simulink model "springDampMass"  (R2021a)
settings: Solver=VariableStepAuto  StartTime=0.0  StopTime=10  FixedStep=10^-2  RelTol=1e-3
model workspace (MAT data in the model file):
  K = 497.616525424
  M = 5
  d = 20.1947463768
libraries: fl_lib x12, nesl_utility x5
settings Model: EnablePacing=on  PacingRate=0.500000  Creator=ditde  LastModifiedBy=ditde

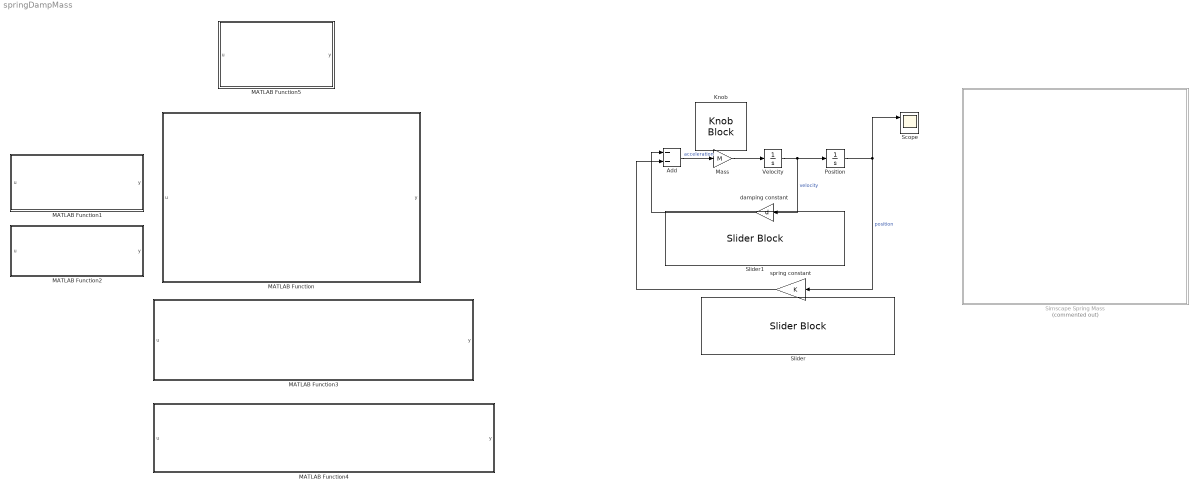
== system springDampMass ==
  Add : Sum  Inputs=--
  Knob : KnobBlock  ScaleMax=5
  MATLAB Function : MATLAB Function  TreatAsAtomicUnit=on
  MATLAB Function1 : MATLAB Function  TreatAsAtomicUnit=on
  MATLAB Function2 : MATLAB Function  TreatAsAtomicUnit=on
  MATLAB Function3 : MATLAB Function  TreatAsAtomicUnit=on
  MATLAB Function4 : MATLAB Function  TreatAsAtomicUnit=on
  MATLAB Function5 : MATLAB Function  TreatAsAtomicUnit=on
  Mass : Gain  Gain=M
  Position : Integrator  InitialCondition=1
  Scope : Scope  NumInputPorts=3
  Simscape Spring Mass : Subsystem  Commented=on
  Slider : SliderBlock  LabelPosition=Bottom  ScaleMax=1000
  Slider1 : SliderBlock  LabelPosition=Hide
  Velocity : Integrator
  damping constant : Gain  Gain=d
  spring constant : Gain  Gain=K
  wires:
  Mass/1 -> Velocity/1
  Velocity/1 -> damping constant/1, Position/1  "velocity"
  Position/1 -> Scope/1, spring constant/1  "position"
  Add/1 -> Mass/1  "acceleration"
  damping constant/1 -> Add/1
  spring constant/1 -> Add/2

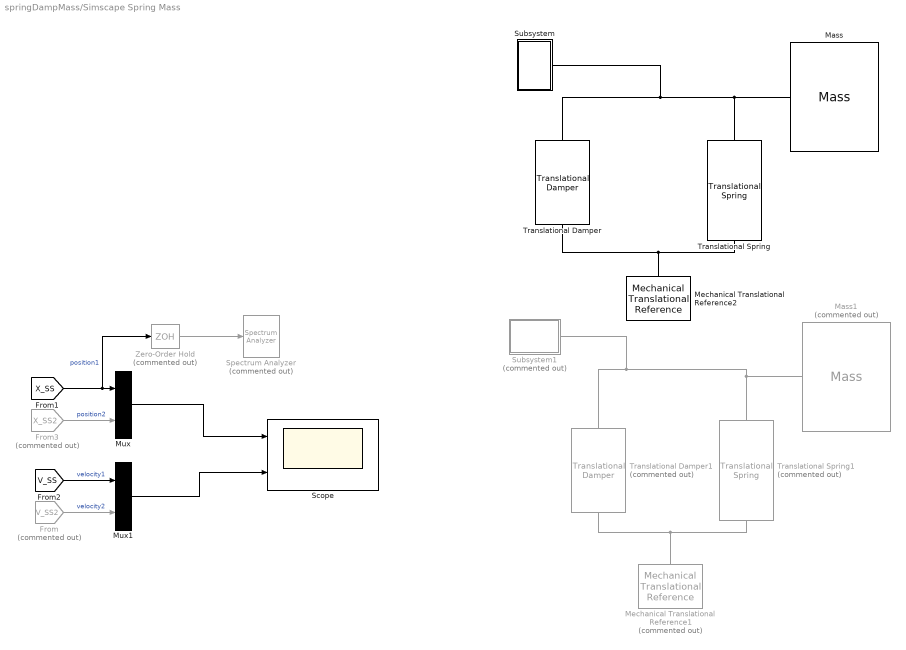
== system springDampMass/Simscape Spring Mass ==
  From : From  Commented=on  GotoTag=V_SS2  TagVisibility=global
  From3 : From  Commented=on  GotoTag=X_SS2  TagVisibility=global
  Mass : fl_lib/Mechanical/Translational Elements/Mass  mass=M kg  num_ports=foundation.enum.numPorts2.one  v_specify=off  v_priority=High  v=0 m/s  v_nominal_specify=off  v_nominal_unit=m/s  v_nominal_value=1  f_specify=off  f_priority=None  f=0 N  f_nominal_specify=off  f_nominal_unit=N  f_nominal_value=1
  Mass1 : fl_lib/Mechanical/Translational Elements/Mass  Commented=on  mass=4.1 kg  num_ports=foundation.enum.numPorts2.one  v_specify=off  v_priority=High  v=0 m/s  v_nominal_specify=off  v_nominal_unit=m/s  v_nominal_value=1  f_specify=off  f_priority=None  f=0 N  f_nominal_specify=off  f_nominal_unit=N  f_nominal_value=1
  Mechanical Translational Reference1 : fl_lib/Mechanical/Translational Elements/Mechanical Translational Reference  Commented=on
  Mechanical Translational Reference2 : fl_lib/Mechanical/Translational Elements/Mechanical Translational Reference
  Mux : Mux  Inputs=2
  Mux1 : Mux  Inputs=2
  Scope : Scope  NumInputPorts=2
  Spectrum Analyzer : SpectrumAnalyzer  Commented=on
  Subsystem : Subsystem
  Subsystem1 : Subsystem  Commented=on
      settings: PortSchema="{\"entries\":[{\"content\":{\"sides\":[{\"content\":{\"connectorIds\":[]},\"type\":\"ConnectorPlacement.EquallySpacedRectSide\",\"uuid\":\"3b3e8523-10d3-43b9-9f77-b9b637dbc56d\"},{\"content\":{\"connectorIds\":[],\"side\":\"RIGHT\"},\"type\":\"ConnectorPlacement.EquallySpacedRectSide\",\"uuid\":\"46eb001f-7b0b-4a31-ad1e-86922fc41839\"},{\"content\":{\"connectorIds\":[],\"side\":\"TOP\"},\"type\":\"ConnectorPlacement.EquallySpacedRectSide\",\"uuid\":\"e7c34988-a452-46fb-a57a-78d1edee4f1a\"},{\"content\":{\"connectorIds\":[\"RConn1\"],\"side\":\"BOTTOM\"},\"type\":\"ConnectorPlacement.EquallySpacedRectSide\",\"uuid\":\"a95b3fbc-c6ac-47a7-9bde-b25b780e38b5\"}]},\"type\":\"ConnectorPlacement.EquallySpacedConnector\",\"uuid\":\"dd414060-0bc3-4aae-86f3-2c1761549555\"}],\"packageUris\":[\"http://schema.mathworks.com/mf0/Connector/R2020b\"],\"version\":\"1.0\"}"
  Translational Damper : fl_lib/Mechanical/Translational Elements/Translational Damper  D=d N/(m/s)  v_specify=off  v_priority=None  v=0 m/s  v_nominal_specify=off  v_nominal_unit=m/s  v_nominal_value=1  f_specify=off  f_priority=None  f=1 N  f_nominal_specify=off  f_nominal_unit=N  f_nominal_value=1
  Translational Damper1 : fl_lib/Mechanical/Translational Elements/Translational Damper  Commented=on  D=0 N/(m/s)  v_specify=off  v_priority=None  v=0 m/s  v_nominal_specify=off  v_nominal_unit=m/s  v_nominal_value=1  f_specify=off  f_priority=None  f=1 N  f_nominal_specify=off  f_nominal_unit=N  f_nominal_value=1
  Translational Spring : fl_lib/Mechanical/Translational Elements/Translational Spring  spr_rate=K N/m  v_specify=off  v_priority=None  v=0 m/s  v_nominal_specify=off  v_nominal_unit=m/s  v_nominal_value=1  f_specify=off  f_priority=None  f=0 N  f_nominal_specify=off  f_nominal_unit=N  f_nominal_value=1  x_specify=on  x_priority=High  x=1 m  x_nominal_specify=off  x_nominal_unit=m  x_nominal_value=1
  Translational Spring1 : fl_lib/Mechanical/Translational Elements/Translational Spring  Commented=on  spr_rate=456 N/m  v_specify=off  v_priority=None  v=0 m/s  v_nominal_specify=off  v_nominal_unit=m/s  v_nominal_value=1  f_specify=off  f_priority=None  f=0 N  f_nominal_specify=off  f_nominal_unit=N  f_nominal_value=1  x_specify=on  x_priority=High  x=1 m  x_nominal_specify=off  x_nominal_unit=m  x_nominal_value=1
  Zero-Order Hold : ZeroOrderHold  Commented=on  SampleTime=-1
  wires:
  [X_SS] -> Zero-Order Hold/1, Mux/1  "position1"
  Zero-Order Hold/1 -> Spectrum Analyzer/1
  Mux/1 -> Scope/1
  From/1 -> Mux1/2  "velocity2"
  From3/1 -> Mux/2  "position2"
  Mux1/1 -> Scope/2
  [V_SS] -> Mux1/1  "velocity1"
  connections:
  Mass1/LConn1 -- Subsystem1/RConn1 -- Translational Damper1/LConn1 -- Translational Spring1/LConn1
  Mass/LConn1 -- Translational Damper/LConn1 -- Subsystem/LConn1 -- Translational Spring/LConn1
  Translational Damper1/RConn1 -- Translational Spring1/RConn1 -- Mechanical Translational Reference1/LConn1
  Translational Damper/RConn1 -- Mechanical Translational Reference2/LConn1 -- Translational Spring/RConn1

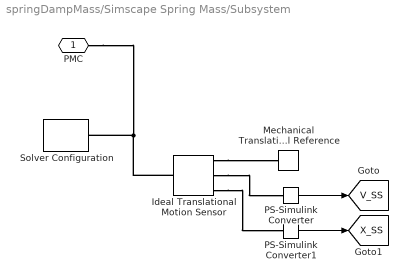
== system springDampMass/Simscape Spring Mass/Subsystem ==
  Ideal Translational Motion Sensor : fl_lib/Mechanical/Mechanical Sensors/Ideal Translational Motion Sensor  offset=1 m
  Mechanical Translational Reference : fl_lib/Mechanical/Translational Elements/Mechanical Translational Reference
  PS-Simulink Converter : nesl_utility/PS-Simulink Converter  PhysicalDomain=network_engine_domain  SubClassName=ps_output  LeftPortType=input  RightPortType=output  PseudoPeriodic=off  Frequencies=[]  Unit=inherit  AffineConversion=off
      settings: SourceProductBaseCode=PW,SS
  PS-Simulink Converter1 : nesl_utility/PS-Simulink Converter  PhysicalDomain=network_engine_domain  SubClassName=ps_output  LeftPortType=input  RightPortType=output  PseudoPeriodic=off  Frequencies=[]  Unit=inherit  AffineConversion=off
      settings: SourceProductBaseCode=PW,SS
  Solver Configuration : nesl_utility/Solver Configuration  PhysicalDomain=network_engine_domain  SubClassName=solver  LeftPortType=input  RightPortType=generic  Tones=[]  Harmonics=[]  SimulateNoise=off  Profile=off  UseLocalSampling=off  EnableSwitchedLinearOptims=on  FrequencyDomain=off  UseCCode=off  RelTol=0.001  AbsTol=1e-06  MinStep=1e-09  ToWorkspace=off  RevertToSquareIcSolve=off  NumHomotopyIterations=100  PhasorMode=off  PhasorModeNumHarmonics=1  DoDC=off  ResidualTolerance=1e-09  UseLocalSolver=off  LocalSolverChoice=NE_BACKWARD_EULER_ADVANCER  LocalSolverSampleTime=0.001  DoFixedCost=off  MaxNonlinIter=3  MaxModeIter=2  ComputeImpulses=off  ImpulseIterations=2  LinearAlgebra=auto  EquationFormulation=NE_TIME_EF  DelaysMemoryBudget=1024  AutomaticFiltering=on  FilteringTimeConstant=0.001  PartitionStorageMethod=AS_NEEDED  PartitionMemoryBudget=1024  PartitionMethod=ROBUST
      settings: SourceProductBaseCode=PW,SS
  PMC : PMIOPort  Side=Left
  tag scope: V_SS=global, X_SS=global
  wires:
  PS-Simulink Converter1/1 -> [X_SS]
  PS-Simulink Converter/1 -> [V_SS]
  connections:
  Ideal Translational Motion Sensor/RConn1 -- Mechanical Translational Reference/LConn1
  Ideal Translational Motion Sensor/LConn1 -- PMC/RConn1 -- Solver Configuration/RConn1
  Ideal Translational Motion Sensor/RConn3 -- PS-Simulink Converter1/LConn1
  Ideal Translational Motion Sensor/RConn2 -- PS-Simulink Converter/LConn1

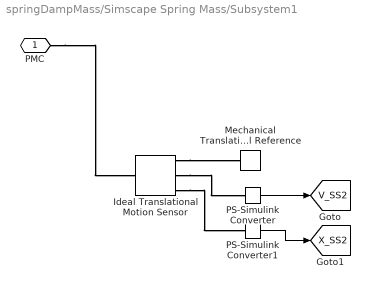
== system springDampMass/Simscape Spring Mass/Subsystem1 ==
  Ideal Translational Motion Sensor : fl_lib/Mechanical/Mechanical Sensors/Ideal Translational Motion Sensor  offset=1 m
  Mechanical Translational Reference : fl_lib/Mechanical/Translational Elements/Mechanical Translational Reference
  PS-Simulink Converter : nesl_utility/PS-Simulink Converter  PhysicalDomain=network_engine_domain  SubClassName=ps_output  LeftPortType=input  RightPortType=output  PseudoPeriodic=off  Frequencies=[]  Unit=inherit  AffineConversion=off
      settings: SourceProductBaseCode=PW,SS
  PS-Simulink Converter1 : nesl_utility/PS-Simulink Converter  PhysicalDomain=network_engine_domain  SubClassName=ps_output  LeftPortType=input  RightPortType=output  PseudoPeriodic=off  Frequencies=[]  Unit=inherit  AffineConversion=off
      settings: SourceProductBaseCode=PW,SS
  PMC : PMIOPort  Side=Right
  tag scope: V_SS2=global, X_SS2=global
  wires:
  PS-Simulink Converter1/1 -> [X_SS2]
  PS-Simulink Converter/1 -> [V_SS2]
  connections:
  Ideal Translational Motion Sensor/RConn1 -- Mechanical Translational Reference/LConn1
  PMC/RConn1 -- Ideal Translational Motion Sensor/LConn1
  Ideal Translational Motion Sensor/RConn3 -- PS-Simulink Converter1/LConn1
  Ideal Translational Motion Sensor/RConn2 -- PS-Simulink Converter/LConn1

== matlab function springDampMass/MATLAB Function ==
  data: u input; y output
function y = fcn(u)

y = u;

== matlab function springDampMass/MATLAB Function2 ==
  data: u input; y output
function y = fcn(u)

y = u;

== matlab function springDampMass/MATLAB Function3 ==
  data: u input; y output
function y = fcn(u)

y = u;

== matlab function springDampMass/MATLAB Function4 ==
  data: u input; y output
function y = fcn(u)

y = u;

== matlab function springDampMass/MATLAB Function5 ==
  data: u input; y output
function y = fcn(u)

y = u;

== matlab function springDampMass/MATLAB Function1 ==
  data: u input; y output
function y = fcn(u)

y = u;
